simulink model "port_checker_2015B"  (R2015b)
settings: Solver=VariableStepAuto  StartTime=0.0  StopTime=10  RelTol=1e-3
libraries: dspnetwork x8, sldrtlib x1
settings Model: Creator=dave  LastModifiedBy=Anony

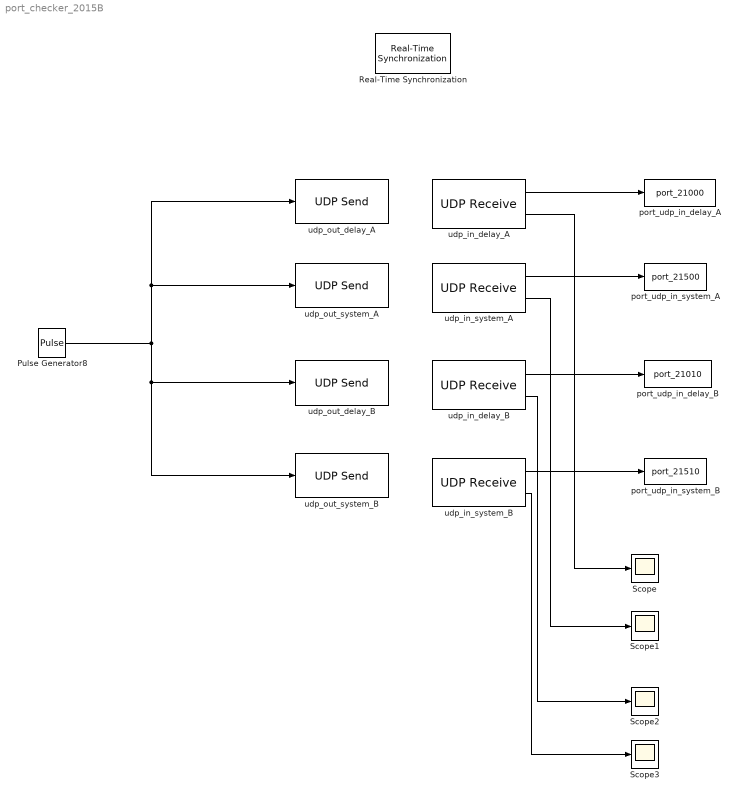
== system port_checker_2015B ==
  Pulse Generator8 : DiscretePulseGenerator  PulseType=Time based  Period=1  PulseWidth=5
  Real-Time Synchronization : sldrtlib/Real-Time Synchronization  SampleTime=0.1  MaxMissedTicks=inf  ShowMissedTicks=off  YieldWhenWaiting=off
  Scope{,1..3} (4 alike) : Scope
  port_udp_in_delay_A : ToWorkspace  VariableName=port_21000  SaveFormat=Timeseries  SampleTime=-1
  port_udp_in_delay_B : ToWorkspace  VariableName=port_21010  SaveFormat=Timeseries  SampleTime=-1
  port_udp_in_system_A : ToWorkspace  VariableName=port_21500  SaveFormat=Timeseries  SampleTime=-1
  port_udp_in_system_B : ToWorkspace  VariableName=port_21510  SaveFormat=Timeseries  SampleTime=-1
  udp_in_delay_A : dspnetwork/UDP Receive  localURL='0.0.0.0'  localPort=21000  remoteURL='127.0.0.1'  remotePort=-1  recvBufferSize=8192  dims=255  signalDatatype=int8  isVarSize=off  showBlockingTime=off  blockingTime=0  sampletime=0.1
  udp_in_delay_B : dspnetwork/UDP Receive  localURL='0.0.0.0'  localPort=21010  remoteURL='127.0.0.1'  remotePort=-1  recvBufferSize=8192  dims=255  signalDatatype=int8  isVarSize=off  showBlockingTime=off  blockingTime=0  sampletime=0.1
  udp_in_system_A : dspnetwork/UDP Receive  localURL='0.0.0.0'  localPort=21500  remoteURL='127.0.0.1'  remotePort=-1  recvBufferSize=8192  dims=255  signalDatatype=int8  isVarSize=off  showBlockingTime=off  blockingTime=0  sampletime=0.1
  udp_in_system_B : dspnetwork/UDP Receive  localURL='0.0.0.0'  localPort=21510  remoteURL='127.0.0.1'  remotePort=-1  recvBufferSize=8192  dims=255  signalDatatype=int8  isVarSize=off  showBlockingTime=off  blockingTime=0  sampletime=0.1
  udp_out_delay_A : dspnetwork/UDP Send  remoteURL='127.0.0.1'  remotePort=20000  localURL='0.0.0.0'  localPortSource=Automatically determine  localPort=-1  sampletime=-1  separateLengthPort=0
  udp_out_delay_B : dspnetwork/UDP Send  remoteURL='127.0.0.1'  remotePort=20010  localURL='0.0.0.0'  localPortSource=Automatically determine  localPort=-1  sampletime=-1  separateLengthPort=0
  udp_out_system_A : dspnetwork/UDP Send  remoteURL='127.0.0.1'  remotePort=20500  localURL='0.0.0.0'  localPortSource=Automatically determine  localPort=-1  sampletime=-1  separateLengthPort=0
  udp_out_system_B : dspnetwork/UDP Send  remoteURL='127.0.0.1'  remotePort=20510  localURL='0.0.0.0'  localPortSource=Automatically determine  localPort=-1  sampletime=-1  separateLengthPort=0
  wires:
  Pulse Generator8/1 -> udp_out_system_B/1, udp_out_delay_B/1, udp_out_system_A/1, udp_out_delay_A/1
  udp_in_delay_A/1 -> port_udp_in_delay_A/1
  udp_in_system_B/1 -> port_udp_in_system_B/1
  udp_in_delay_B/1 -> port_udp_in_delay_B/1
  udp_in_system_A/1 -> port_udp_in_system_A/1
  udp_in_delay_A/2 -> Scope/1
  udp_in_system_A/2 -> Scope1/1
  udp_in_delay_B/2 -> Scope2/1
  udp_in_system_B/2 -> Scope3/1
